simulink model "D_ajsmt"  (R2022b)
settings: Solver=VariableStepAuto  StartTime=0.0  StopTime=800  RelTol=1e-3
settings Model: Creator=Crapon  LastModifiedBy=Crapon

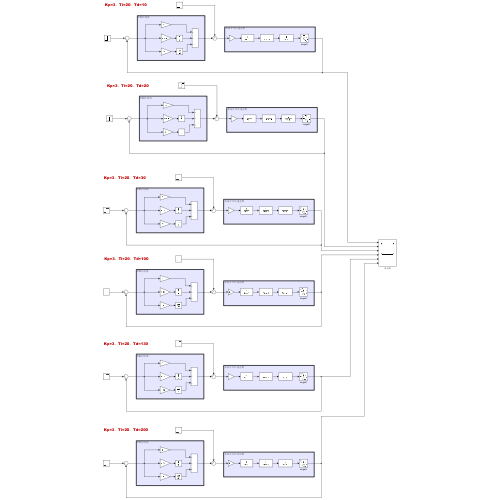
[thumbnail: Simulink's stored preview of the top-level diagram]
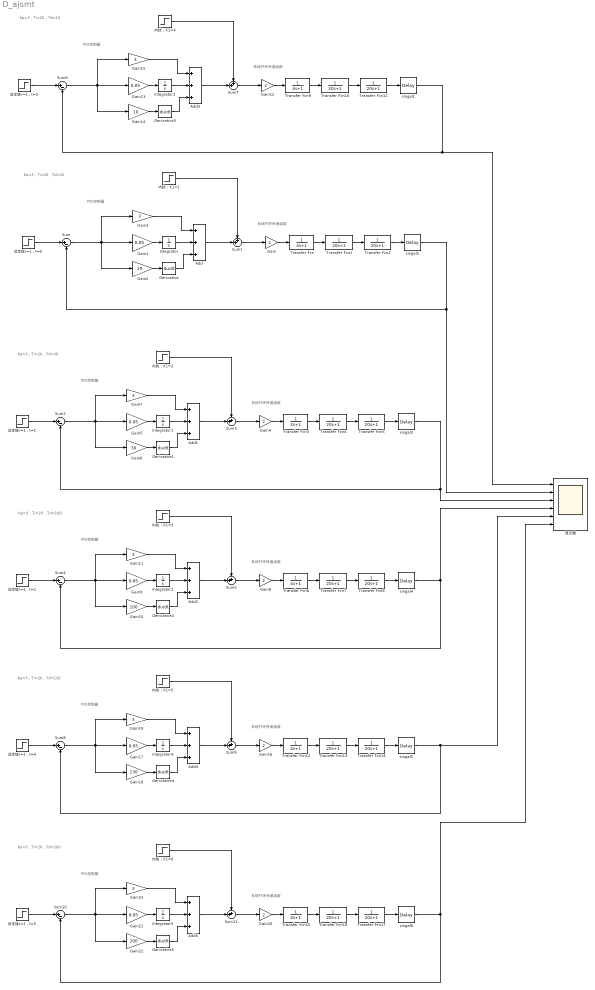
== system D_ajsmt ==
  note: Kp=3，Ti=20，Td=20
  note: PID控制器
  note: 系统开环传递函数
  note: PID控制器
  note: Kp=3，Ti=20，Td=30
  note: 系统开环传递函数
  note: PID控制器
  note: Kp=3，Ti=20，Td=100
  note: 系统开环传递函数
  note: PID控制器
  note: Kp=3，Ti=20，Td=10
  note: 系统开环传递函数
  note: PID控制器
  note: Kp=3，Ti=20，Td=130
  note: 系统开环传递函数
  note: Kp=3，Ti=20，Td=200
  note: PID控制器
  note: 系统开环传递函数
  Add{,1..5} (6 alike) : Sum  Inputs=+++
  Derivative{,1..5} (6 alike) : Derivative
  Gain{,4,8,12,16,20} (6 alike) : Gain  Gain=2
  Gain{1,5,9,13,17,21} (6 alike) : Gain  Gain=0.05
  Gain10 : Gain  Gain=100
  Gain{3,7,11,15,19,23} (6 alike) : Gain  Gain=3
  Gain14 : Gain  Gain=10
  Gain18 : Gain  Gain=130
  Gain2 : Gain  Gain=20
  Gain22 : Gain  Gain=200
  Gain6 : Gain  Gain=30
  Integrator{,1..5} (6 alike) : Integrator
  Sum{,2,4,6,8,10} (6 alike) : Sum  Inputs=|+-
  Sum{1,3,5,7,9,11} (6 alike) : Sum  Inputs=++|
  Transfer Fcn{,3,6,9,12,15} (6 alike) : TransferFcn  Denominator=[4 1]
  Transfer Fcn{1..2,4..5,7..8,10..11,13..14,16..17} (12 alike) : TransferFcn  Denominator=[20 1]
  singal{1..6} (6 alike) : TransportDelay  DelayTime=0
  内扰：X1={1..6} (6 alike) : Step  Time=400  SampleTime=0
  显示器 : Scope  NumInputPorts=6
  设定值r=1，t={0..5} (6 alike) : Step  SampleTime=0
  wires:
  设定值r=1，t=0/1 -> Sum/1
  Transfer Fcn/1 -> Transfer Fcn1/1
  Transfer Fcn1/1 -> Transfer Fcn2/1
  Gain/1 -> Transfer Fcn/1
  Gain1/1 -> Integrator/1
  Gain2/1 -> Derivative/1
  Sum/1 -> Gain2/1, Gain3/1, Gain1/1
  Gain3/1 -> Add/1
  Integrator/1 -> Add/2
  Derivative/1 -> Add/3
  Transfer Fcn2/1 -> singal2/1
  Add/1 -> Sum1/2
  Sum1/1 -> Gain/1
  内扰：X1=1/1 -> Sum1/1
  singal2/1 -> Sum/2, 显示器/2
  singal3/1 -> Sum2/2, 显示器/3
  Sum3/1 -> Gain4/1
  内扰：X1=2/1 -> Sum3/1
  Transfer Fcn4/1 -> Transfer Fcn5/1
  Transfer Fcn5/1 -> singal3/1
  Sum2/1 -> Gain6/1, Gain7/1, Gain5/1
  Derivative1/1 -> Add1/3
  Gain7/1 -> Add1/1
  Gain4/1 -> Transfer Fcn3/1
  Transfer Fcn3/1 -> Transfer Fcn4/1
  Integrator1/1 -> Add1/2
  设定值r=1，t=1/1 -> Sum2/1
  Add1/1 -> Sum3/2
  Gain5/1 -> Integrator1/1
  Gain6/1 -> Derivative1/1
  singal4/1 -> Sum4/2, 显示器/4
  Sum5/1 -> Gain8/1
  内扰：X1=3/1 -> Sum5/1
  Transfer Fcn7/1 -> Transfer Fcn8/1
  Transfer Fcn8/1 -> singal4/1
  Sum4/1 -> Gain10/1, Gain11/1, Gain9/1
  Derivative2/1 -> Add2/3
  Gain11/1 -> Add2/1
  Gain8/1 -> Transfer Fcn6/1
  Transfer Fcn6/1 -> Transfer Fcn7/1
  Integrator2/1 -> Add2/2
  设定值r=1，t=2/1 -> Sum4/1
  Add2/1 -> Sum5/2
  Gain9/1 -> Integrator2/1
  Gain10/1 -> Derivative2/1
  singal1/1 -> 显示器/1, Sum6/2
  Sum7/1 -> Gain12/1
  内扰：X1=4/1 -> Sum7/1
  Transfer Fcn10/1 -> Transfer Fcn11/1
  Transfer Fcn11/1 -> singal1/1
  Sum6/1 -> Gain14/1, Gain15/1, Gain13/1
  Derivative3/1 -> Add3/3
  Gain15/1 -> Add3/1
  Gain12/1 -> Transfer Fcn9/1
  Transfer Fcn9/1 -> Transfer Fcn10/1
  Integrator3/1 -> Add3/2
  设定值r=1，t=3/1 -> Sum6/1
  Add3/1 -> Sum7/2
  Gain13/1 -> Integrator3/1
  Gain14/1 -> Derivative3/1
  singal5/1 -> Sum8/2, 显示器/5
  Sum9/1 -> Gain16/1
  内扰：X1=5/1 -> Sum9/1
  Transfer Fcn13/1 -> Transfer Fcn14/1
  Transfer Fcn14/1 -> singal5/1
  Sum8/1 -> Gain18/1, Gain19/1, Gain17/1
  Derivative4/1 -> Add4/3
  Gain19/1 -> Add4/1
  Gain16/1 -> Transfer Fcn12/1
  Transfer Fcn12/1 -> Transfer Fcn13/1
  Integrator4/1 -> Add4/2
  设定值r=1，t=4/1 -> Sum8/1
  Add4/1 -> Sum9/2
  Gain17/1 -> Integrator4/1
  Gain18/1 -> Derivative4/1
  Gain21/1 -> Integrator5/1
  Sum10/1 -> Gain22/1, Gain23/1, Gain21/1
  Gain22/1 -> Derivative5/1
  Transfer Fcn16/1 -> Transfer Fcn17/1
  Transfer Fcn15/1 -> Transfer Fcn16/1
  Integrator5/1 -> Add5/2
  设定值r=1，t=5/1 -> Sum10/1
  Derivative5/1 -> Add5/3
  singal6/1 -> 显示器/6, Sum10/2
  Gain20/1 -> Transfer Fcn15/1
  Add5/1 -> Sum11/2
  Gain23/1 -> Add5/1
  内扰：X1=6/1 -> Sum11/1
  Transfer Fcn17/1 -> singal6/1
  Sum11/1 -> Gain20/1
